simulink model "MotorCtrl_FOC_Math"  (R2025b)
settings: Solver=FixedStepDiscrete  StartTime=0.0  StopTime=5  FixedStep=MC_Sim_BaseStep  RelTol=1e-3  EnableMultiTasking=on
values from neighbouring files (symbols this model uses):
  MC_ADC_BitNum = 0.0    [MotorControlDataDictionary_Math.sldd]
  MC_ADC_Offset = 0.0    [MotorControlDataDictionary_Math.sldd]
  MC_ADC_VRef = 1.0    [MotorControlDataDictionary_Math.sldd]
  MC_CSA_Gain = 1.0    [MotorControlDataDictionary_Math.sldd]
  MC_MOS_DeadTime = 1.3E-6    [MotorControlDataDictionary_Math.sldd]
  MC_Motor_Mechinal_Damp = 1.0E-5    [MotorControlDataDictionary_Math.sldd]
  MC_Motor_Mechinal_Fric = 0.0    [MotorControlDataDictionary_Math.sldd]
  MC_Motor_Mechinal_Inertia = 0.0103    [MotorControlDataDictionary_Math.sldd]
  MC_Motor_Phi = 0.0059190254913385806    [MotorControlDataDictionary_Math.sldd]
  MC_Motor_Rotor_Pn = 4.0    [MotorControlDataDictionary_Math.sldd]
  MC_Motor_Stator_Ld = 5.6345E-5    [MotorControlDataDictionary_Math.sldd]
  MC_Motor_Stator_Lq = 5.6345E-5    [MotorControlDataDictionary_Math.sldd]
  MC_Motor_Stator_Rs = 0.0286    [MotorControlDataDictionary_Math.sldd]
  MC_Param_CurrentPI_Ki = 0.0089705790612839825    [MotorControlDataDictionary_Math.sldd]
  MC_Param_CurrentPI_Kp = 0.283220860906427    [MotorControlDataDictionary_Math.sldd]
  MC_Param_CurrentPI_UdInteMax = 7.794228634059948    [MotorControlDataDictionary_Math.sldd]
  MC_Param_CurrentPI_UdInteMin = -7.794228634059948    [MotorControlDataDictionary_Math.sldd]
  MC_Param_CurrentPI_UdMax = 7.794228634059948    [MotorControlDataDictionary_Math.sldd]
  MC_Param_CurrentPI_UdMin = -7.794228634059948    [MotorControlDataDictionary_Math.sldd]
  MC_Param_CurrentPI_UqInteMax = 7.794228634059948    [MotorControlDataDictionary_Math.sldd]
  MC_Param_CurrentPI_UqInteMin = -7.794228634059948    [MotorControlDataDictionary_Math.sldd]
  MC_Param_CurrentPI_UqMax = 7.794228634059948    [MotorControlDataDictionary_Math.sldd]
  MC_Param_CurrentPI_UqMin = -7.794228634059948    [MotorControlDataDictionary_Math.sldd]
  MC_Param_Flux_Gamma = 750000.0    [MotorControlDataDictionary_Math.sldd]
  MC_Param_Flux_Lalpha = 5.6345E-5    [MotorControlDataDictionary_Math.sldd]
  MC_Param_Flux_Lbeta = 5.6345E-5    [MotorControlDataDictionary_Math.sldd]
  MC_Param_Flux_Ralpha = 0.0286    [MotorControlDataDictionary_Math.sldd]
  MC_Param_Flux_Rbeta = 0.0286    [MotorControlDataDictionary_Math.sldd]
  MC_Param_Luen_BEMFalpha = -17747.803709290976    [MotorControlDataDictionary_Math.sldd]
  MC_Param_Luen_BEMFbeta = -17747.803709290976    [MotorControlDataDictionary_Math.sldd]
  MC_Param_Luen_BEMFErr = 10.0    [MotorControlDataDictionary_Math.sldd]
  MC_Param_Luen_Currentalpha = -507.58718608572195    [MotorControlDataDictionary_Math.sldd]
  MC_Param_Luen_Currentbeta = -507.58718608572195    [MotorControlDataDictionary_Math.sldd]
  MC_Param_Luen_CurrentErr = 400.0    [MotorControlDataDictionary_Math.sldd]
  MC_Param_Luen_PLL_Ki = 0.24634532585119037    [MotorControlDataDictionary_Math.sldd]
  MC_Param_Luen_PLL_Kp = 125.66370614359172    [MotorControlDataDictionary_Math.sldd]
  MC_Param_Luen_Voltagealpha = 17747.803709290976    [MotorControlDataDictionary_Math.sldd]
  MC_Param_Luen_Voltagebeta = 17747.803709290976    [MotorControlDataDictionary_Math.sldd]
  MC_Param_PhasetoReal = 500.0    [MotorControlDataDictionary_Math.sldd]
  MC_Param_SMO_CoffA = 0.968326559588251    [MotorControlDataDictionary_Math.sldd]
  MC_Param_SMO_CoffB = 1.1074629514597569    [MotorControlDataDictionary_Math.sldd]
  MC_Param_SpeedCtrl_IdMax = 60.0    [MotorControlDataDictionary_Math.sldd]
  MC_Param_SpeedCtrl_IdMin = -60.0    [MotorControlDataDictionary_Math.sldd]
  MC_Param_SpeedCtrl_IqMax = 60.0    [MotorControlDataDictionary_Math.sldd]
  MC_Param_SpeedCtrl_IqMin = -60.0    [MotorControlDataDictionary_Math.sldd]
  MC_Param_SpeedPI_Ki = 0.57157085739428382    [MotorControlDataDictionary_Math.sldd]
  MC_Param_SpeedPI_Kp = 9.1114109857344836    [MotorControlDataDictionary_Math.sldd]
  MC_Param_SpeedtoTheta = 6.24E-5    [MotorControlDataDictionary_Math.sldd]
  MC_Param_SVPWM_DutyMax = 0.98    [MotorControlDataDictionary_Math.sldd]
  MC_Param_SVPWM_DutyMin = 0.02    [MotorControlDataDictionary_Math.sldd]
  MC_Param_SVPWM_SampleOffset1 = 0.02    [MotorControlDataDictionary_Math.sldd]
  MC_Param_SVPWM_SampleOffset2 = 0.015    [MotorControlDataDictionary_Math.sldd]
  MC_Param_SVPWM_SampleValid = 0.0096153846153846159    [MotorControlDataDictionary_Math.sldd]
  MC_Param_Zero = 0.0    [MotorControlDataDictionary_Math.sldd]
  MC_Sample_CurrentNoise = 1.0E-15    [MotorControlDataDictionary_Math.sldd]
  MC_Sample_Rs = 0.002    [MotorControlDataDictionary_Math.sldd]
  MC_Sample_VbusNoise = 1.0E-15    [MotorControlDataDictionary_Math.sldd]
  MC_Sim_BaseStep = 2.08E-8    [MotorControlDataDictionary_Math.sldd]
  MC_Sim_HFTStep = 6.24E-5    [MotorControlDataDictionary_Math.sldd]
  MC_Sim_MFTStep = 0.0019968    [MotorControlDataDictionary_Math.sldd]
libraries: simulink x28, nesl_utility x19, fl_lib x14, ee_lib x13, autolibpmsminterior x2, autolibinverter x1
(part 7 of 8)

== system MotorCtrl_FOC_Math/Hardware_Sim/currentSample/getCurrentSample_TRS(Three) ==
  SampleTrigger : Inport
  Current : Inport  Port=2
  Demux : Demux  Outputs=3
  Mux : Mux  Inputs=3
  getCurrentSampleA : Subsystem  TreatAsAtomicUnit=on
  getCurrentSampleB : Subsystem  TreatAsAtomicUnit=on
  getCurrentSampleC : Subsystem  TreatAsAtomicUnit=on
  SampleCurrent : Outport
  wires:
  getCurrentSampleA/1(SampleCurrentA) -> Mux/1
  getCurrentSampleB/1(SampleCurrentB) -> Mux/2
  Mux/1 -> SampleCurrent/1
  getCurrentSampleC/1(SampleCurrentC) -> Mux/3
  SampleTrigger/1 -> getCurrentSampleB/Trigger, getCurrentSampleC/Trigger, getCurrentSampleA/Trigger
  Current/1 -> Demux/1
  Demux/1 -> getCurrentSampleA/1(Current)
  Demux/2 -> getCurrentSampleB/1(Current)
  Demux/3 -> getCurrentSampleC/1(Current)

== system MotorCtrl_FOC_Math/Hardware_Sim/currentSample/getCurrentSample_TRS(Two) ==
  SampleTrigger : Inport
  Current : Inport  Port=2
  Demux : Demux  Outputs=2
  Mux : Mux  Inputs=2
  getCurrentSample1 : Subsystem  TreatAsAtomicUnit=on
  getCurrentSample2 : Subsystem  TreatAsAtomicUnit=on
  SampleCurrent : Outport
  wires:
  Demux/1 -> getCurrentSample1/Trigger
  Current/1 -> getCurrentSample2/1(Current), getCurrentSample1/1(Current)
  Demux/2 -> getCurrentSample2/Trigger
  getCurrentSample1/1(SampleCurrentUp) -> Mux/1
  getCurrentSample2/1(SampleCurrentDown) -> Mux/2
  Mux/1 -> SampleCurrent/1
  SampleTrigger/1 -> Demux/1

== system MotorCtrl_FOC_Math/MFTask/adrcofSpeed/ESO ==
  SpeedReal : Inport
  u : Inport  Port=2
  Add : Sum  Inputs=+-+
  Add1 : Sum
  Delay One Step : Delay  DelayLength=1  InitialCondition=MC_Param_Zero
  Subsystem : Subsystem
  Subsystem1 : Subsystem
  Subtract : Sum  Inputs=+-
  b : Gain  Gain=3*MC_Motor_Rotor_Pn*MC_Motor_Phi/(2*MC_Motor_Mechinal_Inertia)  ParamDataTypeStr=single  OutDataTypeStr=single  RndMeth=Simplest
  z1 : Outport
  z2 : Outport  Port=2
  wires:
  u/1 -> b/1
  SpeedReal/1 -> Subtract/2
  Subtract/1 -> Subsystem/1(In1), Subsystem1/1(In1)  "Err_ESO"
  Add/1 -> Add1/1
  Add1/1 -> z1/1, Delay One Step/1
  Delay One Step/1 -> Add1/2, [z1_ESO_Delay]
  Subsystem/1(Out1) -> Add/2
  b/1 -> Add/3
  [z1_ESO_Delay] -> Subtract/1
  Subsystem1/1(z2) -> Add/1, z2/1

== system MotorCtrl_FOC_Math/MFTask/adrcofSpeed/LESO ==
  Id : Inport
  Ud : Inport  Port=2
  Iq : Inport  Port=3
  Uq : Inport  Port=4
  Add1 : Sum  Inputs=+++  AccumDataTypeStr=single  RndMeth=Simplest
  Add{2,4..6} (4 alike) : Sum
  Add3 : Sum  Inputs=+++  AccumDataTypeStr=single  RndMeth=Simplest
  Constant : Constant  Value=0.5  OutDataTypeStr=single
  Constant1 : Constant  Value=0.5  OutDataTypeStr=single
  Constant2 : Constant  Value=MC_Sim_HFTStep*10  OutDataTypeStr=single
  Constant3 : Constant  Value=MC_Sim_HFTStep*10  OutDataTypeStr=single
  Delay{,1..3} (4 alike) : Delay  DelayLength=1  InitialCondition=single(0)
  Gain{,1,3..4} (4 alike) : Gain
  Gain2 : Gain  Gain=1/2
  Gain5 : Gain  Gain=1/2
  Gain6 : Gain  Gain=1/single(MC_Motor_Stator_Ld)
  Gain7 : Gain  Gain=1/single(MC_Motor_Stator_Lq)
  Subtract1 : Sum  Inputs=+-
  Subtract2 : Sum  Inputs=+-
  Ts{1..4} (4 alike) : Gain  Gain=single(MC_Sim_HFTStep)  ParamDataTypeStr=single  OutDataTypeStr=single  RndMeth=Simplest
  falFunc : Subsystem
  falFunc1 : Subsystem
  falFunc2 : Subsystem
  falFunc3 : Subsystem
  Id_ESO : Outport
  Iq_ESO : Outport  Port=2
  Id_Dis : Outport  Port=3
  Iq_Dis : Outport  Port=4
  wires:
  [Id_ESO_Delay] -> Subtract1/2
  Subtract1/1 -> falFunc1/1(Err), falFunc/1(Err)  "Ed"
  Id/1 -> Subtract1/1
  falFunc/1(FalOutput) -> Gain/1  "Id_ESO_F1"
  Gain/1 -> Add3/2
  Ud/1 -> Gain6/1
  Add3/1 -> Ts1/1
  Ts1/1 -> Add4/1
  Add4/1 -> Delay/1, Id_ESO/1  "Id_ESO"
  Delay/1 -> Add4/2, [Id_ESO_Delay]
  falFunc1/1(FalOutput) -> Gain1/1  "Id_ESO_F2"
  Add5/1 -> Id_Dis/1, Delay1/1, Add3/3  "Id_Dis"
  Gain1/1 -> Ts2/1
  Ts2/1 -> Add5/1
  Delay1/1 -> Add5/2
  Constant/1 -> Gain2/1, falFunc/2(Alpha)
  Gain2/1 -> falFunc1/2(Alpha)
  Gain5/1 -> falFunc3/2(Alpha)
  Constant1/1 -> falFunc2/2(Alpha), Gain5/1
  Delay3/1 -> Add6/2
  Ts4/1 -> Add6/1
  Gain4/1 -> Ts4/1
  Add6/1 -> Add1/3, Iq_Dis/1, Delay3/1  "Iq_Dis"
  falFunc3/1(FalOutput) -> Gain4/1  "Iq_ESO_F2"
  Delay2/1 -> [Iq_ESO_Delay], Add2/2
  Add2/1 -> Iq_ESO/1, Delay2/1  "Iq_ESO"
  Ts3/1 -> Add2/1
  Add1/1 -> Ts3/1
  Uq/1 -> Gain7/1
  Gain3/1 -> Add1/2
  falFunc2/1(FalOutput) -> Gain3/1  "Iq_ESO_F1"
  Iq/1 -> Subtract2/1
  Subtract2/1 -> falFunc2/1(Err), falFunc3/1(Err)  "Ed"
  [Iq_ESO_Delay] -> Subtract2/2
  Constant2/1 -> falFunc1/3(Delta), falFunc/3(Delta)
  Constant3/1 -> falFunc2/3(Delta), falFunc3/3(Delta)
  Gain6/1 -> Add3/1
  Gain7/1 -> Add1/1

== system MotorCtrl_FOC_Math/MFTask/adrcofSpeed/NLSEF ==
  " SpeedRef" : Inport
  " z" : Inport  Port=2
  " d" : Inport  Port=3
  Gain : Gain  Gain=(2*MC_Motor_Mechinal_Inertia)/(3*MC_Motor_Rotor_Pn*MC_Motor_Phi)  ParamDataTypeStr=single  OutDataTypeStr=single  RndMeth=Simplest
  Subsystem : Subsystem
  Subtract : Sum  Inputs=+-
  Subtract1 : Sum  Inputs=+-
  IqRef : Outport
  wires:
  " SpeedRef"/1 -> Subtract/1
  " z"/1 -> Subtract/2
  Subtract/1 -> Subsystem/1(In1)  "SpeedErr"
  " d"/1 -> Gain/1
  Subsystem/1(IqRef) -> Subtract1/1
  Gain/1 -> Subtract1/2
  Subtract1/1 -> IqRef/1

== system MotorCtrl_FOC_Math/MFTask/adrcofSpeed/Tracking-Differentiator ==
  Ref_In : Inport
  Add : Sum
  Add1 : Sum
  Delay One Step : Delay  DelayLength=1  InitialCondition=MC_Param_Zero
  Delay One Step1 : Delay  DelayLength=1  InitialCondition=MC_Param_Zero
  Gain : Gain  Gain=MC_Sim_MFTStep  ParamDataTypeStr=single  OutDataTypeStr=single  RndMeth=Simplest
  Gain1 : Gain  Gain=MC_Sim_MFTStep  OutDataTypeStr=single  RndMeth=Simplest
  Signal Copy : SignalConversion  OverrideOpt=off
  Subsystem : Subsystem
  SpeedTarget_TD : Outport
  wires:
  Ref_In/1 -> Subsystem/1(Ref_In)
  Subsystem/1(Ref_TD) -> Gain/1  "u"
  Add/1 -> Gain1/1, Delay One Step/1  "x2"
  Delay One Step/1 -> Add/2, [x2_delay]
  Gain/1 -> Add/1  "T*u"
  Gain1/1 -> Add1/1  "T*x2"
  Add1/1 -> Signal Copy/1, Delay One Step1/1  "x1"
  Delay One Step1/1 -> Add1/2, [x1_delay]
  Signal Copy/1 -> SpeedTarget_TD/1  "SpeedTarget_TD"
  [x1_delay] -> Subsystem/2(X1)
  [x2_delay] -> Subsystem/3(X2)

== system MotorCtrl_FOC_Math/HFTask/currentADRC/LESO/falFunc ==
  Err : Inport
  Alpha : Inport  Port=2
  Delta : Inport  Port=3
  Abs : Abs  SaturateOnIntegerOverflow=off
  Constant : Constant  OutDataTypeStr=single
  Divide : Product  Inputs=*/  OutDataTypeStr=single  RndMeth=Simplest
  Math Function : Math  Operator=pow  OutputSignalType=real
  Math Function1 : Math  Operator=pow  OutputSignalType=real
  Product : Product  OutDataTypeStr=single  RndMeth=Simplest
  Relational Operator : RelationalOperator  Operator=<=  OutDataTypeStr=boolean  RndMeth=Simplest  InputSameDT=off
  Sign : Signum
  Subtract : Sum  Inputs=+-
  Switch : Switch  Criteria=u2 > Threshold  SaturateOnIntegerOverflow=off  InputSameDT=off
  FalOutput : Outport
  wires:
  Switch/1 -> FalOutput/1
  Product/1 -> Switch/3
  Sign/1 -> Product/2
  Math Function1/1 -> Product/1
  Alpha/1 -> Subtract/2, Math Function1/2
  Divide/1 -> Switch/1
  Constant/1 -> Subtract/1
  Subtract/1 -> Math Function/2
  Math Function/1 -> Divide/2
  Relational Operator/1 -> Switch/2
  Delta/1 -> Relational Operator/2, Math Function/1
  Abs/1 -> Relational Operator/1, Math Function1/1
  Err/1 -> Abs/1, Sign/1, Divide/1

== system MotorCtrl_FOC_Math/HFTask/svpwm/getVoltageExchange/getSectorN ==
  Valpha : Inport
  Vbeta : Inport  Port=2
  Add : Sum
  Add1 : Sum  Inputs=+++
  Constant : Constant
  Constant1 : Constant  Value=0
  Gain : Gain  Gain=sqrt(3)/2
  Gain1 : Gain  Gain=-1/2
  Gain2 : Gain
  Gain3 : Gain  Gain=2
  Gain4 : Gain  Gain=4
  Subtract : Sum  Inputs=-+
  Switch : Switch  Criteria=u2 > Threshold  SaturateOnIntegerOverflow=off  InputSameDT=off
  Switch1 : Switch  Criteria=u2 > Threshold  SaturateOnIntegerOverflow=off  InputSameDT=off
  Switch2 : Switch  Criteria=u2 > Threshold  SaturateOnIntegerOverflow=off  InputSameDT=off
  SectorN : Outport
  wires:
  Constant/1 -> Switch1/1, Switch/1, Switch2/1
  Gain3/1 -> Add1/2
  Gain1/1 -> Add/2, Subtract/2
  Switch/1 -> Gain2/1
  Gain/1 -> Add/1, Subtract/1
  Switch1/1 -> Gain3/1
  Vbeta/1 -> Switch/2, Gain1/1  "U1"
  Constant1/1 -> Switch2/3, Switch1/3, Switch/3
  Valpha/1 -> Gain/1
  Subtract/1 -> Switch2/2  "U3"
  Gain2/1 -> Add1/3
  Switch2/1 -> Gain4/1
  Add/1 -> Switch1/2  "U2"
  Gain4/1 -> Add1/1
  Add1/1 -> SectorN/1  "SectorN"

== system MotorCtrl_FOC_Math/Hardware_Math/PWMGenerate/DeadTimeGenerate/APhaseDeadTime ==
  FLag : Inport
  AH : Inport  Port=2
  AL : Inport  Port=3
  DeadTime : Inport  Port=4
  Add : Sum
  Subtract : Sum  Inputs=+-
  Switch : Switch  Criteria=u2 > Threshold  SaturateOnIntegerOverflow=off  InputSameDT=off
  Switch1 : Switch  Criteria=u2 > Threshold  SaturateOnIntegerOverflow=off  InputSameDT=off
  ADH : Outport
  ADL : Outport  Port=2
  wires:
  DeadTime/1 -> Add/2, Subtract/2
  AL/1 -> Switch/3, Subtract/1
  FLag/1 -> Switch/2, Switch1/2
  Add/1 -> Switch/1
  Switch/1 -> ADH/1  "ADH"
  AH/1 -> Switch1/1, Add/1
  Subtract/1 -> Switch1/3
  Switch1/1 -> ADL/1  "ADL"

== system MotorCtrl_FOC_Math/Hardware_Math/PWMGenerate/DeadTimeGenerate/BPhaseDeadTime ==
  FLag : Inport
  BH : Inport  Port=2
  BL : Inport  Port=3
  DeadTime : Inport  Port=4
  Add : Sum
  Subtract : Sum  Inputs=+-
  Switch : Switch  Criteria=u2 > Threshold  SaturateOnIntegerOverflow=off  InputSameDT=off
  Switch1 : Switch  Criteria=u2 > Threshold  SaturateOnIntegerOverflow=off  InputSameDT=off
  BDH : Outport
  BDL : Outport  Port=2
  wires:
  Switch1/1 -> BDL/1  "BDL"
  Subtract/1 -> Switch1/3
  BH/1 -> Switch1/1, Add/1
  Switch/1 -> BDH/1  "BDH"
  Add/1 -> Switch/1
  FLag/1 -> Switch1/2, Switch/2
  BL/1 -> Subtract/1, Switch/3
  DeadTime/1 -> Subtract/2, Add/2

== system MotorCtrl_FOC_Math/Hardware_Math/PWMGenerate/DeadTimeGenerate/CPhaseDeadTime ==
  FLag : Inport
  CH : Inport  Port=2
  CL : Inport  Port=3
  DeadTime : Inport  Port=4
  Add : Sum
  Subtract : Sum  Inputs=+-
  Switch : Switch  Criteria=u2 > Threshold  SaturateOnIntegerOverflow=off  InputSameDT=off
  Switch1 : Switch  Criteria=u2 > Threshold  SaturateOnIntegerOverflow=off  InputSameDT=off
  CDH : Outport
  CDL : Outport  Port=2
  wires:
  DeadTime/1 -> Add/2, Subtract/2
  CL/1 -> Switch/3, Subtract/1
  FLag/1 -> Switch/2, Switch1/2
  Add/1 -> Switch/1
  Switch/1 -> CDH/1  "CDH"
  CH/1 -> Switch1/1, Add/1
  Subtract/1 -> Switch1/3
  Switch1/1 -> CDL/1  "CDL"

== system MotorCtrl_FOC_Math/Hardware_Math/currentSample/getCurrentSample_ORS_Double/getCurrentSample1 ==
  Current : Inport
  Trigger : TriggerPort  VariantControl=(inherit)
  ADCOffset : Constant  Value=MC_ADC_Offset  SampleTime=-1
  ADCQuality : Gain  Gain=2^MC_ADC_BitNum/MC_ADC_VRef
  Add : Sum
  CSAGain : Gain  Gain=MC_CSA_Gain
  Data Type Conversion3 : DataTypeConversion  OutDataTypeStr=single  SaturateOnIntegerOverflow=off  RndMeth=Floor
  SampleCurrentUp : Outport
  wires:
  ADCQuality/1 -> Data Type Conversion3/1
  ADCOffset/1 -> Add/1
  Add/1 -> ADCQuality/1
  CSAGain/1 -> Add/2
  Data Type Conversion3/1 -> SampleCurrentUp/1  "SampleCurrentUp"
  Current/1 -> CSAGain/1

== system MotorCtrl_FOC_Math/Hardware_Math/currentSample/getCurrentSample_ORS_Double/getCurrentSample2 ==
  Current : Inport
  Trigger : TriggerPort  TriggerType=falling  VariantControl=(inherit)
  ADCOffset : Constant  Value=MC_ADC_Offset  SampleTime=-1
  ADCQuality : Gain  Gain=2^MC_ADC_BitNum/MC_ADC_VRef
  Add : Sum
  CSAGain : Gain  Gain=MC_CSA_Gain
  Data Type Conversion3 : DataTypeConversion  OutDataTypeStr=single  SaturateOnIntegerOverflow=off  RndMeth=Floor
  SampleCurrentDown : Outport
  wires:
  Current/1 -> CSAGain/1
  Add/1 -> ADCQuality/1
  Data Type Conversion3/1 -> SampleCurrentDown/1  "SampleCurrentDown"
  ADCOffset/1 -> Add/1
  ADCQuality/1 -> Data Type Conversion3/1
  CSAGain/1 -> Add/2

== system MotorCtrl_FOC_Math/Hardware_Math/currentSample/getCurrentSample_ORS_Single/getCurrentSample1 ==
  Current : Inport
  Trigger : TriggerPort  VariantControl=(inherit)
  ADCOffset : Constant  Value=0  SampleTime=-1
  ADCQuality : Gain
  Add : Sum
  CSAGain : Gain
  Data Type Conversion3 : DataTypeConversion  OutDataTypeStr=single  SaturateOnIntegerOverflow=off  RndMeth=Floor
  SampleCurrentUp : Outport
  wires:
  ADCQuality/1 -> Data Type Conversion3/1
  ADCOffset/1 -> Add/1
  Add/1 -> ADCQuality/1
  CSAGain/1 -> Add/2
  Data Type Conversion3/1 -> SampleCurrentUp/1  "SampleCurrentUp"
  Current/1 -> CSAGain/1

== system MotorCtrl_FOC_Math/Hardware_Math/currentSample/getCurrentSample_ORS_Single/getCurrentSample2 ==
  Current : Inport
  Trigger : TriggerPort  VariantControl=(inherit)
  ADCOffset : Constant  Value=0  SampleTime=-1
  ADCQuality : Gain
  Add : Sum
  CSAGain : Gain
  Data Type Conversion3 : DataTypeConversion  OutDataTypeStr=single  SaturateOnIntegerOverflow=off  RndMeth=Floor
  SampleCurrentDown : Outport
  wires:
  Current/1 -> CSAGain/1
  CSAGain/1 -> Add/2
  Add/1 -> ADCQuality/1
  ADCOffset/1 -> Add/1
  ADCQuality/1 -> Data Type Conversion3/1
  Data Type Conversion3/1 -> SampleCurrentDown/1  "SampleCurrentDown"

== system MotorCtrl_FOC_Math/Hardware_Math/currentSample/getCurrentSample_TRS(Three)/getCurrentSampleA ==
  Current : Inport
  Trigger : TriggerPort  TriggerType=falling  VariantControl=(inherit)
  ADCOffset : Constant  Value=0  SampleTime=-1
  ADCQuality : Gain
  Add : Sum
  CSAGain : Gain
  Data Type Conversion3 : DataTypeConversion  OutDataTypeStr=single  SaturateOnIntegerOverflow=off  RndMeth=Floor
  SampleCurrentA : Outport
  wires:
  ADCQuality/1 -> Data Type Conversion3/1
  ADCOffset/1 -> Add/1
  Add/1 -> ADCQuality/1
  CSAGain/1 -> Add/2
  Data Type Conversion3/1 -> SampleCurrentA/1  "SampleCurrentA"
  Current/1 -> CSAGain/1

== system MotorCtrl_FOC_Math/Hardware_Math/currentSample/getCurrentSample_TRS(Three)/getCurrentSampleB ==
  Current : Inport
  Trigger : TriggerPort  TriggerType=falling  VariantControl=(inherit)
  ADCOffset : Constant  Value=0  SampleTime=-1
  ADCQuality : Gain
  Add : Sum
  CSAGain : Gain
  Data Type Conversion3 : DataTypeConversion  OutDataTypeStr=single  SaturateOnIntegerOverflow=off  RndMeth=Floor
  SampleCurrentB : Outport
  wires:
  Current/1 -> CSAGain/1
  Data Type Conversion3/1 -> SampleCurrentB/1  "SampleCurrentB"
  CSAGain/1 -> Add/2
  Add/1 -> ADCQuality/1
  ADCOffset/1 -> Add/1
  ADCQuality/1 -> Data Type Conversion3/1

== system MotorCtrl_FOC_Math/Hardware_Math/currentSample/getCurrentSample_TRS(Three)/getCurrentSampleC ==
  Current : Inport
  Trigger : TriggerPort  TriggerType=falling  VariantControl=(inherit)
  ADCOffset : Constant  Value=0  SampleTime=-1
  ADCQuality : Gain
  Add : Sum
  CSAGain : Gain
  Data Type Conversion3 : DataTypeConversion  OutDataTypeStr=single  SaturateOnIntegerOverflow=off  RndMeth=Floor
  SampleCurrentC : Outport
  wires:
  ADCQuality/1 -> Data Type Conversion3/1
  ADCOffset/1 -> Add/1
  Add/1 -> ADCQuality/1
  CSAGain/1 -> Add/2
  Data Type Conversion3/1 -> SampleCurrentC/1  "SampleCurrentC"
  Current/1 -> CSAGain/1

== system MotorCtrl_FOC_Math/Hardware_Math/currentSample/getCurrentSample_TRS(Two)/getCurrentSample1 ==
  Current : Inport
  Trigger : TriggerPort  VariantControl=(inherit)
  ADCOffset : Constant  Value=0  SampleTime=-1
  ADCQuality : Gain
  Add : Sum
  CSAGain : Gain
  Data Type Conversion3 : DataTypeConversion  OutDataTypeStr=single  SaturateOnIntegerOverflow=off  RndMeth=Floor
  SampleCurrentUp : Outport
  wires:
  ADCQuality/1 -> Data Type Conversion3/1
  ADCOffset/1 -> Add/1
  Add/1 -> ADCQuality/1
  CSAGain/1 -> Add/2
  Data Type Conversion3/1 -> SampleCurrentUp/1  "SampleCurrentUp"
  Current/1 -> CSAGain/1

== system MotorCtrl_FOC_Math/Hardware_Math/currentSample/getCurrentSample_TRS(Two)/getCurrentSample2 ==
  Current : Inport
  Trigger : TriggerPort  TriggerType=falling  VariantControl=(inherit)
  ADCOffset : Constant  Value=0  SampleTime=-1
  ADCQuality : Gain
  Add : Sum
  CSAGain : Gain
  Data Type Conversion3 : DataTypeConversion  OutDataTypeStr=single  SaturateOnIntegerOverflow=off  RndMeth=Floor
  SampleCurrentDown : Outport
  wires:
  Current/1 -> CSAGain/1
  Data Type Conversion3/1 -> SampleCurrentDown/1  "SampleCurrentDown"
  CSAGain/1 -> Add/2
  Add/1 -> ADCQuality/1
  ADCOffset/1 -> Add/1
  ADCQuality/1 -> Data Type Conversion3/1

== system MotorCtrl_FOC_Math/Hardware_Sim/PWMGenerate/DeadTimeGenerate/APhaseDeadTime ==
  FLag : Inport
  AH : Inport  Port=2
  AL : Inport  Port=3
  DeadTime : Inport  Port=4
  Add : Sum
  Subtract : Sum  Inputs=+-
  Switch : Switch  Criteria=u2 > Threshold  SaturateOnIntegerOverflow=off  InputSameDT=off
  Switch1 : Switch  Criteria=u2 > Threshold  SaturateOnIntegerOverflow=off  InputSameDT=off
  ADH : Outport
  ADL : Outport  Port=2
  wires:
  DeadTime/1 -> Add/2, Subtract/2
  AL/1 -> Switch/3, Subtract/1
  FLag/1 -> Switch/2, Switch1/2
  Add/1 -> Switch/1
  Switch/1 -> ADH/1  "ADH"
  AH/1 -> Switch1/1, Add/1
  Subtract/1 -> Switch1/3
  Switch1/1 -> ADL/1  "ADL"

== system MotorCtrl_FOC_Math/Hardware_Sim/PWMGenerate/DeadTimeGenerate/BPhaseDeadTime ==
  FLag : Inport
  BH : Inport  Port=2
  BL : Inport  Port=3
  DeadTime : Inport  Port=4
  Add : Sum
  Subtract : Sum  Inputs=+-
  Switch : Switch  Criteria=u2 > Threshold  SaturateOnIntegerOverflow=off  InputSameDT=off
  Switch1 : Switch  Criteria=u2 > Threshold  SaturateOnIntegerOverflow=off  InputSameDT=off
  BDH : Outport
  BDL : Outport  Port=2
  wires:
  Switch1/1 -> BDL/1  "BDL"
  Subtract/1 -> Switch1/3
  BH/1 -> Switch1/1, Add/1
  Switch/1 -> BDH/1  "BDH"
  Add/1 -> Switch/1
  FLag/1 -> Switch1/2, Switch/2
  BL/1 -> Subtract/1, Switch/3
  DeadTime/1 -> Subtract/2, Add/2

== system MotorCtrl_FOC_Math/Hardware_Sim/PWMGenerate/DeadTimeGenerate/CPhaseDeadTime ==
  FLag : Inport
  CH : Inport  Port=2
  CL : Inport  Port=3
  DeadTime : Inport  Port=4
  Add : Sum
  Subtract : Sum  Inputs=+-
  Switch : Switch  Criteria=u2 > Threshold  SaturateOnIntegerOverflow=off  InputSameDT=off
  Switch1 : Switch  Criteria=u2 > Threshold  SaturateOnIntegerOverflow=off  InputSameDT=off
  CDH : Outport
  CDL : Outport  Port=2
  wires:
  DeadTime/1 -> Add/2, Subtract/2
  CL/1 -> Switch/3, Subtract/1
  FLag/1 -> Switch/2, Switch1/2
  Add/1 -> Switch/1
  Switch/1 -> CDH/1  "CDH"
  CH/1 -> Switch1/1, Add/1
  Subtract/1 -> Switch1/3
  Switch1/1 -> CDL/1  "CDL"

== system MotorCtrl_FOC_Math/Hardware_Sim/currentSample/getCurrentSample_ORS_Double/getCurrentSample1 ==
  Current : Inport
  Trigger : TriggerPort  VariantControl=(inherit)
  ADCOffset : Constant  Value=MC_ADC_Offset  SampleTime=-1
  ADCQuality : Gain  Gain=2^MC_ADC_BitNum/MC_ADC_VRef
  Add : Sum
  CSAGain : Gain  Gain=MC_CSA_Gain
  Data Type Conversion3 : DataTypeConversion  OutDataTypeStr=single  SaturateOnIntegerOverflow=off  RndMeth=Floor
  SampleCurrentUp : Outport
  wires:
  ADCQuality/1 -> Data Type Conversion3/1
  ADCOffset/1 -> Add/1
  Add/1 -> ADCQuality/1
  CSAGain/1 -> Add/2
  Data Type Conversion3/1 -> SampleCurrentUp/1  "SampleCurrentUp"
  Current/1 -> CSAGain/1

== system MotorCtrl_FOC_Math/Hardware_Sim/currentSample/getCurrentSample_ORS_Double/getCurrentSample2 ==
  Current : Inport
  Trigger : TriggerPort  TriggerType=falling  VariantControl=(inherit)
  ADCOffset : Constant  Value=MC_ADC_Offset  SampleTime=-1
  ADCQuality : Gain  Gain=2^MC_ADC_BitNum/MC_ADC_VRef
  Add : Sum
  CSAGain : Gain  Gain=MC_CSA_Gain
  Data Type Conversion3 : DataTypeConversion  OutDataTypeStr=single  SaturateOnIntegerOverflow=off  RndMeth=Floor
  SampleCurrentDown : Outport
  wires:
  Current/1 -> CSAGain/1
  Add/1 -> ADCQuality/1
  Data Type Conversion3/1 -> SampleCurrentDown/1  "SampleCurrentDown"
  ADCOffset/1 -> Add/1
  ADCQuality/1 -> Data Type Conversion3/1
  CSAGain/1 -> Add/2

== system MotorCtrl_FOC_Math/Hardware_Sim/currentSample/getCurrentSample_ORS_Single/getCurrentSample1 ==
  Current : Inport
  Trigger : TriggerPort  VariantControl=(inherit)
  ADCOffset : Constant  Value=0  SampleTime=-1
  ADCQuality : Gain
  Add : Sum
  CSAGain : Gain
  Data Type Conversion3 : DataTypeConversion  OutDataTypeStr=single  SaturateOnIntegerOverflow=off  RndMeth=Floor
  SampleCurrentUp : Outport
  wires:
  ADCQuality/1 -> Data Type Conversion3/1
  ADCOffset/1 -> Add/1
  Add/1 -> ADCQuality/1
  CSAGain/1 -> Add/2
  Data Type Conversion3/1 -> SampleCurrentUp/1  "SampleCurrentUp"
  Current/1 -> CSAGain/1

== system MotorCtrl_FOC_Math/Hardware_Sim/currentSample/getCurrentSample_ORS_Single/getCurrentSample2 ==
  Current : Inport
  Trigger : TriggerPort  VariantControl=(inherit)
  ADCOffset : Constant  Value=0  SampleTime=-1
  ADCQuality : Gain
  Add : Sum
  CSAGain : Gain
  Data Type Conversion3 : DataTypeConversion  OutDataTypeStr=single  SaturateOnIntegerOverflow=off  RndMeth=Floor
  SampleCurrentDown : Outport
  wires:
  Current/1 -> CSAGain/1
  CSAGain/1 -> Add/2
  Add/1 -> ADCQuality/1
  ADCOffset/1 -> Add/1
  ADCQuality/1 -> Data Type Conversion3/1
  Data Type Conversion3/1 -> SampleCurrentDown/1  "SampleCurrentDown"

== system MotorCtrl_FOC_Math/Hardware_Sim/currentSample/getCurrentSample_TRS(Three)/getCurrentSampleA ==
  Current : Inport
  Trigger : TriggerPort  TriggerType=falling  VariantControl=(inherit)
  ADCOffset : Constant  Value=0  SampleTime=-1
  ADCQuality : Gain
  Add : Sum
  CSAGain : Gain
  Data Type Conversion3 : DataTypeConversion  OutDataTypeStr=single  SaturateOnIntegerOverflow=off  RndMeth=Floor
  SampleCurrentA : Outport
  wires:
  ADCQuality/1 -> Data Type Conversion3/1
  ADCOffset/1 -> Add/1
  Add/1 -> ADCQuality/1
  CSAGain/1 -> Add/2
  Data Type Conversion3/1 -> SampleCurrentA/1  "SampleCurrentA"
  Current/1 -> CSAGain/1

== system MotorCtrl_FOC_Math/Hardware_Sim/currentSample/getCurrentSample_TRS(Three)/getCurrentSampleB ==
  Current : Inport
  Trigger : TriggerPort  TriggerType=falling  VariantControl=(inherit)
  ADCOffset : Constant  Value=0  SampleTime=-1
  ADCQuality : Gain
  Add : Sum
  CSAGain : Gain
  Data Type Conversion3 : DataTypeConversion  OutDataTypeStr=single  SaturateOnIntegerOverflow=off  RndMeth=Floor
  SampleCurrentB : Outport
  wires:
  Current/1 -> CSAGain/1
  Data Type Conversion3/1 -> SampleCurrentB/1  "SampleCurrentB"
  CSAGain/1 -> Add/2
  Add/1 -> ADCQuality/1
  ADCOffset/1 -> Add/1
  ADCQuality/1 -> Data Type Conversion3/1

== system MotorCtrl_FOC_Math/Hardware_Sim/currentSample/getCurrentSample_TRS(Three)/getCurrentSampleC ==
  Current : Inport
  Trigger : TriggerPort  TriggerType=falling  VariantControl=(inherit)
  ADCOffset : Constant  Value=0  SampleTime=-1
  ADCQuality : Gain
  Add : Sum
  CSAGain : Gain
  Data Type Conversion3 : DataTypeConversion  OutDataTypeStr=single  SaturateOnIntegerOverflow=off  RndMeth=Floor
  SampleCurrentC : Outport
  wires:
  ADCQuality/1 -> Data Type Conversion3/1
  ADCOffset/1 -> Add/1
  Add/1 -> ADCQuality/1
  CSAGain/1 -> Add/2
  Data Type Conversion3/1 -> SampleCurrentC/1  "SampleCurrentC"
  Current/1 -> CSAGain/1

== system MotorCtrl_FOC_Math/Hardware_Sim/currentSample/getCurrentSample_TRS(Two)/getCurrentSample1 ==
  Current : Inport
  Trigger : TriggerPort  VariantControl=(inherit)
  ADCOffset : Constant  Value=0  SampleTime=-1
  ADCQuality : Gain
  Add : Sum
  CSAGain : Gain
  Data Type Conversion3 : DataTypeConversion  OutDataTypeStr=single  SaturateOnIntegerOverflow=off  RndMeth=Floor
  SampleCurrentUp : Outport
  wires:
  ADCQuality/1 -> Data Type Conversion3/1
  ADCOffset/1 -> Add/1
  Add/1 -> ADCQuality/1
  CSAGain/1 -> Add/2
  Data Type Conversion3/1 -> SampleCurrentUp/1  "SampleCurrentUp"
  Current/1 -> CSAGain/1

== system MotorCtrl_FOC_Math/Hardware_Sim/currentSample/getCurrentSample_TRS(Two)/getCurrentSample2 ==
  Current : Inport
  Trigger : TriggerPort  TriggerType=falling  VariantControl=(inherit)
  ADCOffset : Constant  Value=0  SampleTime=-1
  ADCQuality : Gain
  Add : Sum
  CSAGain : Gain
  Data Type Conversion3 : DataTypeConversion  OutDataTypeStr=single  SaturateOnIntegerOverflow=off  RndMeth=Floor
  SampleCurrentDown : Outport
  wires:
  Current/1 -> CSAGain/1
  Data Type Conversion3/1 -> SampleCurrentDown/1  "SampleCurrentDown"
  CSAGain/1 -> Add/2
  Add/1 -> ADCQuality/1
  ADCOffset/1 -> Add/1
  ADCQuality/1 -> Data Type Conversion3/1

== system MotorCtrl_FOC_Math/MFTask/adrcofSpeed/ESO/Subsystem ==
  In1 : Inport
  Gain : Gain  Gain=2*pi*100
  Out1 : Outport
  wires:
  In1/1 -> Gain/1
  Gain/1 -> Out1/1

== system MotorCtrl_FOC_Math/MFTask/adrcofSpeed/ESO/Subsystem1 ==
  In1 : Inport
  Gain : Gain  Gain=-2*pi*100*2
  z2 : Outport
  wires:
  In1/1 -> Gain/1
  Gain/1 -> z2/1  "z2"

== system MotorCtrl_FOC_Math/MFTask/adrcofSpeed/LESO/falFunc ==
  Err : Inport
  Alpha : Inport  Port=2
  Delta : Inport  Port=3
  Abs : Abs  SaturateOnIntegerOverflow=off
  Constant : Constant  OutDataTypeStr=single
  Divide : Product  Inputs=*/  OutDataTypeStr=single  RndMeth=Simplest
  Math Function : Math  Operator=pow  OutputSignalType=real
  Math Function1 : Math  Operator=pow  OutputSignalType=real
  Product : Product  OutDataTypeStr=single  RndMeth=Simplest
  Relational Operator : RelationalOperator  Operator=<=  OutDataTypeStr=boolean  RndMeth=Simplest  InputSameDT=off
  Sign : Signum
  Subtract : Sum  Inputs=+-
  Switch : Switch  Criteria=u2 > Threshold  SaturateOnIntegerOverflow=off  InputSameDT=off
  FalOutput : Outport
  wires:
  Err/1 -> Divide/1, Sign/1, Abs/1
  Abs/1 -> Math Function1/1, Relational Operator/1
  Delta/1 -> Math Function/1, Relational Operator/2
  Relational Operator/1 -> Switch/2
  Math Function/1 -> Divide/2
  Subtract/1 -> Math Function/2
  Constant/1 -> Subtract/1
  Divide/1 -> Switch/1
  Alpha/1 -> Math Function1/2, Subtract/2
  Math Function1/1 -> Product/1
  Sign/1 -> Product/2
  Product/1 -> Switch/3
  Switch/1 -> FalOutput/1
